simulink model "SimulacionCTRL3"  (R2021b)
settings: Solver=VariableStepAuto  StartTime=0.0  StopTime=20  RelTol=1e-3
undefined symbols (not defined in the file): coefDen, coefNum, kdr, ki, ki2, ki3, kp, kpr
libraries: simulink x2
settings Model: Creator=nicol  LastModifiedBy=CASA

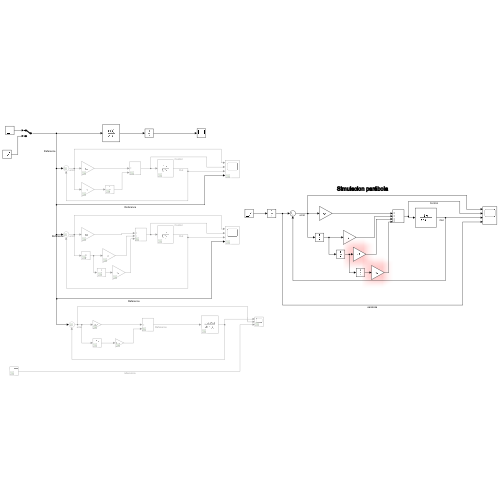
[thumbnail: Simulink's stored preview of the top-level diagram]
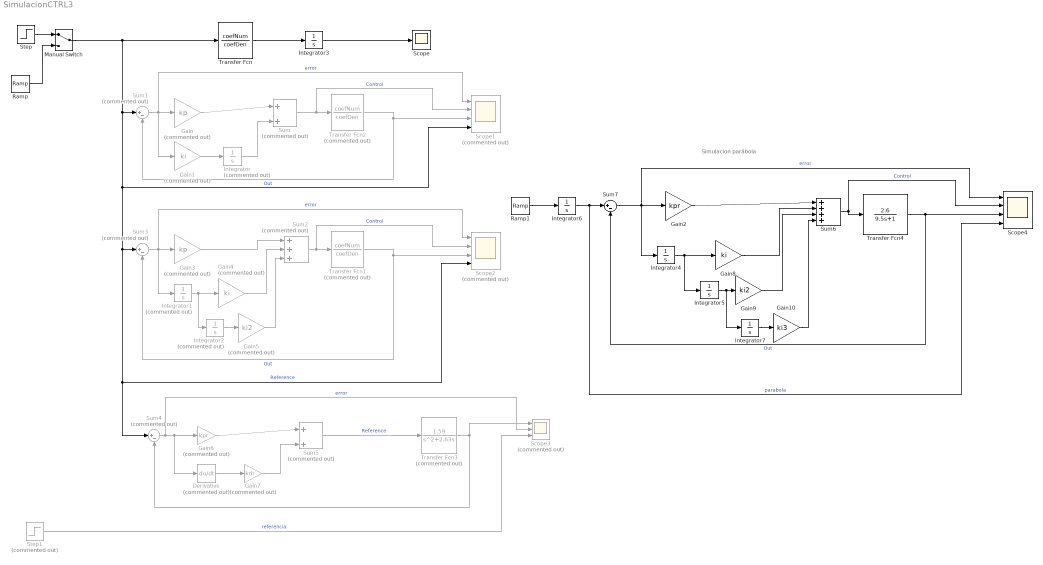
== system SimulacionCTRL3 ==
  note: Simulacion parábola
  Derivative : Derivative  Commented=on
  Gain : Gain  Commented=on  Gain=kp
  Gain1 : Gain  Commented=on  Gain=ki
  Gain10 : Gain  Gain=ki3
  Gain2 : Gain  Gain=kpr
  Gain3 : Gain  Commented=on  Gain=kp
  Gain4 : Gain  Commented=on  Gain=ki
  Gain5 : Gain  Commented=on  Gain=ki2
  Gain6 : Gain  Commented=on  Gain=kpr
  Gain7 : Gain  Commented=on  Gain=kdr
  Gain8 : Gain  Gain=ki
  Gain9 : Gain  Gain=ki2
  Integrator : Integrator  Commented=on
  Integrator1 : Integrator  Commented=on
  Integrator2 : Integrator  Commented=on
  Integrator{3..7} (5 alike) : Integrator
  Manual Switch : ManualSwitch
  Ramp : simulink/Sources/Ramp  slope=1  start=0  InitialOutput=0
  Ramp1 : simulink/Sources/Ramp  slope=1  start=0  InitialOutput=0
  Scope : Scope
  Scope1 : Scope  Commented=on  NumInputPorts=4
  Scope2 : Scope  Commented=on  NumInputPorts=4
  Scope3 : Scope  Commented=on  NumInputPorts=3
  Scope4 : Scope  NumInputPorts=4
  Step : Step  Time=0  SampleTime=0
  Step1 : Step  Commented=on  Time=0  SampleTime=0
  Sum : Sum  Commented=on  Inputs=|++
  Sum1 : Sum  Commented=on  Inputs=|+-
  Sum2 : Sum  Commented=on  Inputs=|+++
  Sum3 : Sum  Commented=on  Inputs=|+-
  Sum4 : Sum  Commented=on  Inputs=|+-
  Sum5 : Sum  Commented=on  Inputs=|++
  Sum6 : Sum  Inputs=|++++
  Sum7 : Sum  Inputs=|+-
  Transfer Fcn : TransferFcn  Numerator=coefNum  Denominator=coefDen
  Transfer Fcn1 : TransferFcn  Commented=on  Numerator=coefNum  Denominator=coefDen
  Transfer Fcn2 : TransferFcn  Commented=on  Numerator=coefNum  Denominator=coefDen
  Transfer Fcn3 : TransferFcn  Commented=on  Numerator=[1.59]  Denominator=[1 2.63 0]
  Transfer Fcn4 : TransferFcn  Numerator=[2.6]  Denominator=[9.5 1]
  wires:
  Gain1/1 -> Integrator/1
  Gain/1 -> Sum/1
  Integrator/1 -> Sum/2
  Sum/1 -> Scope1/2, Transfer Fcn2/1  "Control"
  Sum1/1 -> Gain1/1, Scope1/1, Gain/1  "error"
  Transfer Fcn2/1 -> Scope1/3, Sum1/2  "Out"
  Manual Switch/1 -> Sum3/1, Sum4/1, Scope2/4, Scope1/4, Sum1/1, Transfer Fcn/1  "Reference"
  Transfer Fcn1/1 -> Sum3/2, Scope2/3  "Out"
  Sum3/1 -> Gain3/1, Scope2/1, Integrator1/1  "error"
  Sum2/1 -> Transfer Fcn1/1, Scope2/2  "Control"
  Gain4/1 -> Sum2/2
  Gain3/1 -> Sum2/1
  Integrator1/1 -> Integrator2/1, Gain4/1
  Integrator2/1 -> Gain5/1
  Gain5/1 -> Sum2/3
  Step/1 -> Manual Switch/1
  Ramp/1 -> Manual Switch/2
  Transfer Fcn/1 -> Integrator3/1
  Integrator3/1 -> Scope/1
  Sum4/1 -> Scope3/2, Derivative/1, Gain6/1  "error"
  Derivative/1 -> Gain7/1
  Gain6/1 -> Sum5/1
  Gain7/1 -> Sum5/2
  Transfer Fcn3/1 -> Sum4/2, Scope3/1
  Sum5/1 -> Transfer Fcn3/1  "Reference"
  Step1/1 -> Scope3/3  "referencia"
  Gain9/1 -> Sum6/3
  Integrator5/1 -> Integrator7/1, Gain9/1
  Integrator4/1 -> Gain8/1, Integrator5/1
  Gain2/1 -> Sum6/1
  Gain8/1 -> Sum6/2
  Sum6/1 -> Scope4/2, Transfer Fcn4/1  "Control"
  Sum7/1 -> Integrator4/1, Scope4/1, Gain2/1  "error"
  Transfer Fcn4/1 -> Sum7/2, Scope4/3  "Out"
  Ramp1/1 -> Integrator6/1
  Integrator6/1 -> Scope4/4, Sum7/1  "parabola"
  Integrator7/1 -> Gain10/1
  Gain10/1 -> Sum6/4
